simulink model "PWPF_simple"  (R2021b)
settings: Solver=VariableStepAuto  StartTime=0.0  StopTime=0.6  RelTol=1e-3
values from neighbouring files (symbols this model uses):
  K_m = 4.5    [pwpf_replication.m]    (also in thrustsimpwpf.m)
  K_p = 1    [pwpf_replication.m]    (also in thrustsimpwpf.m)
  T_m = 0.85    [pwpf_replication.m]    (also in thrustsimpwpf.m)
  U_off = U_on/3    (= 0.15)    [pwpf_replication.m]    (also in thrustsimpwpf.m = 0.0888888888889)
  U_on = 0.45    [pwpf_replication.m]    (also in thrustsimpwpf.m = 0.8)
settings Model: Creator=nnatsoul  LastModifiedBy=nnatsoul

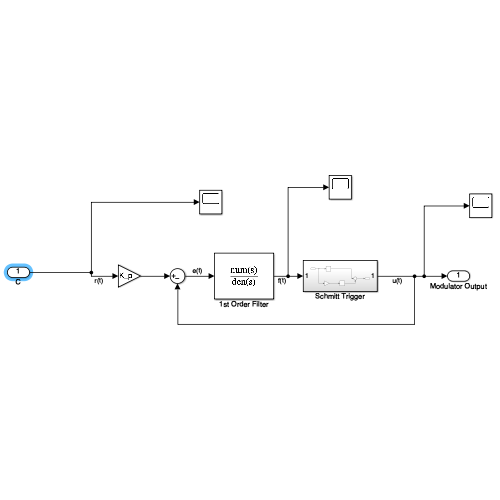
[thumbnail: Simulink's stored preview of the top-level diagram]
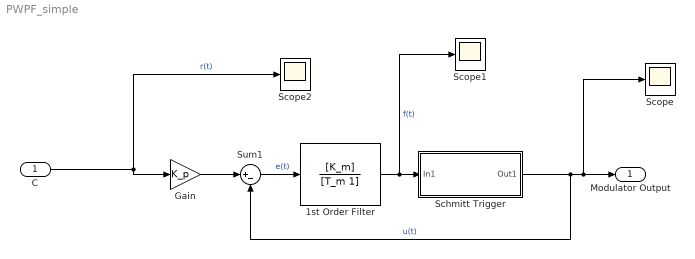
== system PWPF_simple ==
  C : Inport
  1st Order Filter : TransferFcn  Numerator=[K_m]  Denominator=[T_m 1]
  Gain : Gain  Gain=K_p
  Schmitt Trigger : Subsystem
  Scope : Scope
  Scope1 : Scope
  Scope2 : Scope
  Sum1 : Sum  Inputs=|+-
  Modulator Output : Outport
  wires:
  C/1 -> Gain/1, Scope2/1  "r(t)"
  Gain/1 -> Sum1/1
  Sum1/1 -> 1st Order Filter/1  "e(t)"
  1st Order Filter/1 -> Scope1/1, Schmitt Trigger/1(In1)  "f(t)"
  Schmitt Trigger/1(Out1) -> Scope/1, Modulator Output/1, Sum1/2  "u(t)"

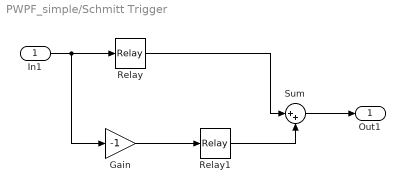
== system PWPF_simple/Schmitt Trigger ==
  In1 : Inport
  Gain : Gain  Gain=-1
  Relay : Relay  OnSwitchValue=U_on  OffSwitchValue=U_off
  Relay1 : Relay  OnSwitchValue=U_on  OffSwitchValue=U_off
  Sum : Sum  Inputs=|++
  Out1 : Outport
  wires:
  In1/1 -> Gain/1, Relay/1
  Relay/1 -> Sum/1
  Relay1/1 -> Sum/2
  Gain/1 -> Relay1/1
  Sum/1 -> Out1/1
